simulink model "test_model_hw_only"  (R2017a)
settings: Solver=FixedStepDiscrete  StartTime=0.0  StopTime=Inf  RelTol=1e-3
libraries: MoDesA_lib x2
settings Model: Creator=streit  LastModifiedBy=streit
settings SolverCC: EnableConcurrentExecution=on  ConcurrentTasks=on

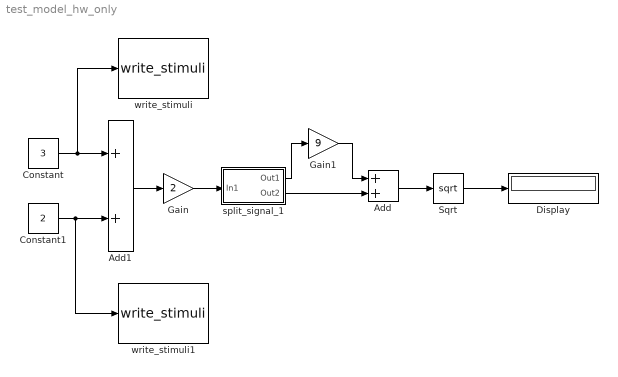
== system test_model_hw_only ==
  Add : Sum  Tag=hw_ip  OutDataTypeStr=uint16
  Add1 : Sum  Tag=hw_ip  OutDataTypeStr=uint16
  Constant : Constant  Value=3  OutDataTypeStr=uint8
  Constant1 : Constant  Value=2  OutDataTypeStr=uint8
  Display : Display
  Gain : Gain  Tag=hw_ip  Gain=2  OutDataTypeStr=uint8
  Gain1 : Gain  Tag=hw_ip  Gain=9  OutDataTypeStr=uint16
  Sqrt : Sqrt  Tag=hw_ip  OutputSignalType=real  OutDataTypeStr=uint8  SaturateOnIntegerOverflow=on
  split_signal_1 : Subsystem  Tag=hw_ip
  write_stimuli : MoDesA_lib/write_stimuli  bound=1  instance=0
      settings: SourceProductName=Custom Lib for MoDesA code generator
  write_stimuli1 : MoDesA_lib/write_stimuli  bound=1  instance=1
      settings: SourceProductName=Custom Lib for MoDesA code generator
  wires:
  Gain1/1 -> Add/1
  split_signal_1/1(Out1) -> Gain1/1
  split_signal_1/2(Out2) -> Add/2
  Sqrt/1 -> Display/1
  Add/1 -> Sqrt/1
  Gain/1 -> split_signal_1/1(In1)
  Constant/1 -> write_stimuli/1, Add1/1
  Constant1/1 -> write_stimuli1/1, Add1/2
  Add1/1 -> Gain/1

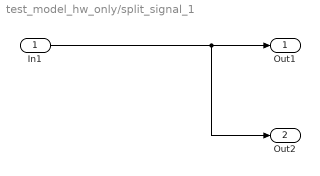
== system test_model_hw_only/split_signal_1 ==
  In1 : Inport
  Out1 : Outport
  Out2 : Outport  Port=2
  wires:
  In1/1 -> Out2/1, Out1/1
